simulink model "FirstPrincValveInjector_AlgebraicLoopOnly_Testing"  (R2025b)
settings: Solver=VariableStepAuto  StartTime=0.0  StopTime=10.0  RelTol=1e-3
undefined symbols (not defined in the file): A_inj_ox, Cd_inj_ox, CdA_table, epsilon, mdot_ox_nom_cstar_match, P_1_ox, P_c_nom, psi_to_Pa, rho_ox, theta_bp
settings Model: Creator=gruby  LastModifiedBy=gruby

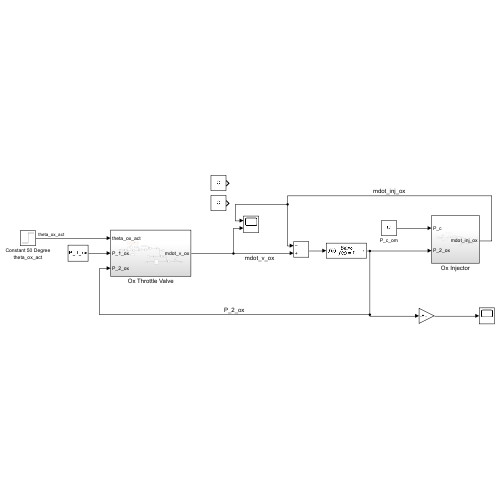
[thumbnail: Simulink's stored preview of the top-level diagram]
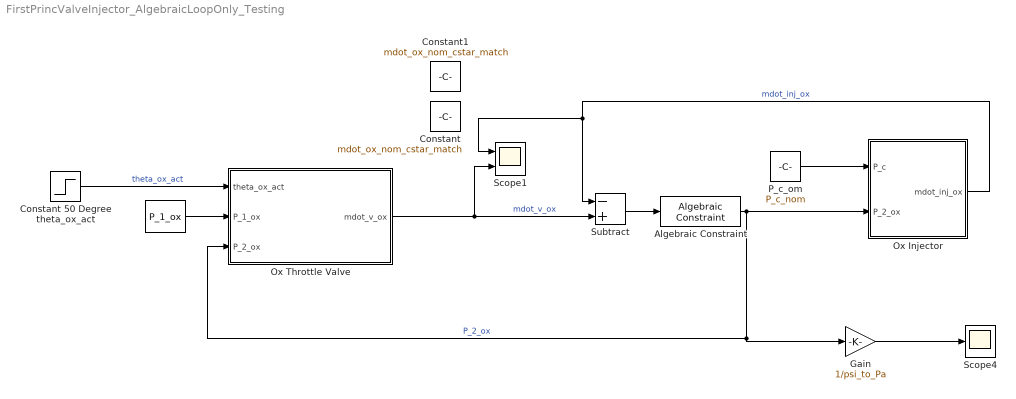
== system FirstPrincValveInjector_AlgebraicLoopOnly_Testing ==
  " " : Constant  Value=P_1_ox
  Algebraic Constraint : AlgebraicConstraint  InitialGuess=P_amb
  Constant : Constant  Value=mdot_ox_nom_cstar_match
  Constant 50 Degree theta_ox_act : Step  Time=10  Before=50  After=50  SampleTime=0
  Constant1 : Constant  Value=mdot_ox_nom_cstar_match
  Gain : Gain  Gain=1/psi_to_Pa
  Ox Injector : Subsystem
  Ox Throttle Valve : Subsystem
  P_c_om : Constant  Value=P_c_nom
  Scope1 : Scope  NumInputPorts=2
      settings: ActiveDisplayYMinimum=-1  ActiveDisplayYMaximum=1  DataLoggingVariableName=ScopeData3
  Scope4 : Scope
      settings: ActiveDisplayYMinimum=299.56325226947473  ActiveDisplayYMaximum=499.56325226947473  DataLoggingVariableName=ScopeData18
  Subtract : Sum  Inputs=-+
  wires:
  Ox Injector/1(mdot_inj_ox) -> Subtract/1, Scope1/1  "mdot_inj_ox"
  " "/1 -> Ox Throttle Valve/2(P_1_ox)
  Ox Throttle Valve/1(mdot_v_ox) -> Scope1/2, Subtract/2  "mdot_v_ox"
  Algebraic Constraint/1 -> Ox Injector/2(P_2_ox), Ox Throttle Valve/3(P_2_ox), Gain/1  "P_2_ox"
  Subtract/1 -> Algebraic Constraint/1
  Constant 50 Degree theta_ox_act/1 -> Ox Throttle Valve/1(theta_ox_act)  "theta_ox_act"
  P_c_om/1 -> Ox Injector/1(P_c)
  Gain/1 -> Scope4/1

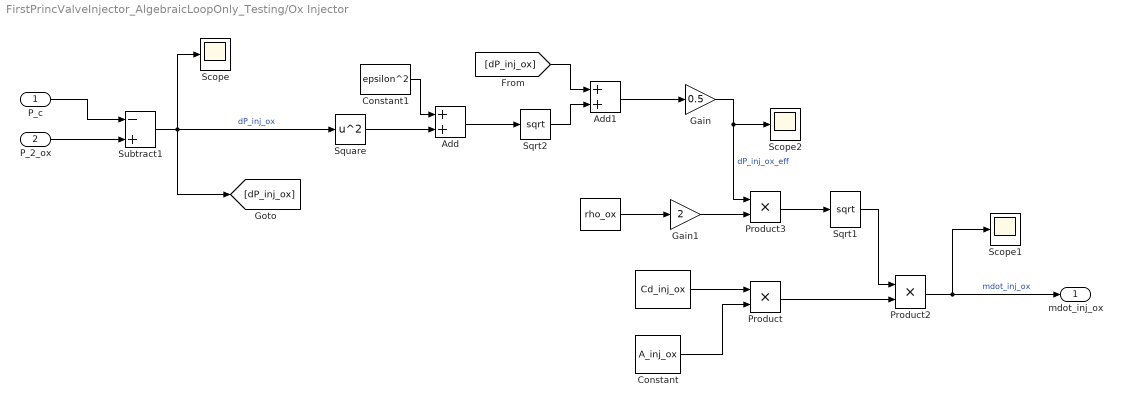
== system FirstPrincValveInjector_AlgebraicLoopOnly_Testing/Ox Injector ==
  P_c : Inport
  P_2_ox : Inport  Port=2
  " " : Constant  Value=rho_ox
  "    " : Constant  Value=Cd_inj_ox
  Add : Sum
  Add1 : Sum
  Constant : Constant  Value=A_inj_ox
  Constant1 : Constant  Value=epsilon^2
  Gain : Gain  Gain=0.5
  Gain1 : Gain  Gain=2
  Product : Product
  Product2 : Product
  Product3 : Product
  Scope : Scope
      settings: ActiveDisplayYMinimum=-1  ActiveDisplayYMaximum=1
  Scope1 : Scope
      settings: ActiveDisplayYMinimum=-1  ActiveDisplayYMaximum=1  DataLoggingVariableName=ScopeData2
  Scope2 : Scope
      settings: DataLoggingVariableName=ScopeData21
  Sqrt1 : Sqrt
  Sqrt2 : Sqrt
  Square : Math  Operator=square
  Subtract1 : Sum  Inputs=-+
  mdot_inj_ox : Outport
  wires:
  Subtract1/1 -> [dP_inj_ox], Square/1, Scope/1  "dP_inj_ox"
  "    "/1 -> Product/1
  " "/1 -> Gain1/1
  P_2_ox/1 -> Subtract1/2
  Product3/1 -> Sqrt1/1
  Sqrt1/1 -> Product2/1
  Gain1/1 -> Product3/2
  P_c/1 -> Subtract1/1
  Product2/1 -> Scope1/1, mdot_inj_ox/1  "mdot_inj_ox"
  Constant/1 -> Product/2
  Product/1 -> Product2/2
  Add1/1 -> Gain/1
  Sqrt2/1 -> Add1/2
  Add/1 -> Sqrt2/1
  [dP_inj_ox] -> Add1/1
  Constant1/1 -> Add/1
  Square/1 -> Add/2
  Gain/1 -> Product3/1, Scope2/1  "dP_inj_ox_eff"

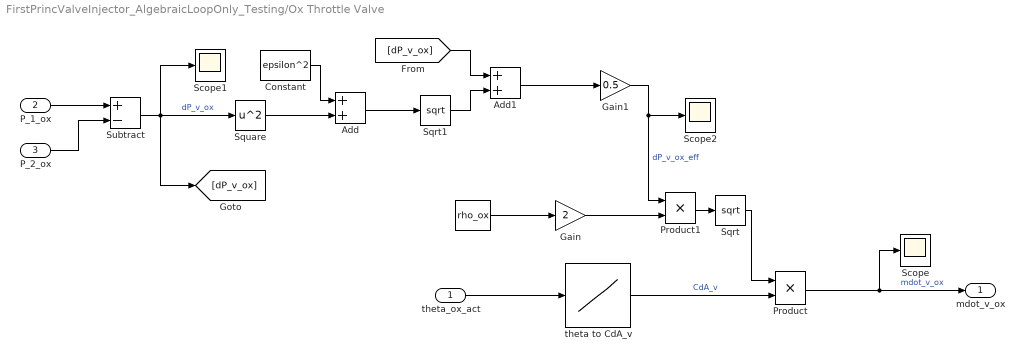
== system FirstPrincValveInjector_AlgebraicLoopOnly_Testing/Ox Throttle Valve ==
  theta_ox_act : Inport
  P_1_ox : Inport  Port=2
  P_2_ox : Inport  Port=3
  "  " : Constant  Value=rho_ox
  Add : Sum
  Add1 : Sum
  Constant : Constant  Value=epsilon^2
  Gain : Gain  Gain=2
  Gain1 : Gain  Gain=0.5
  Product : Product
  Product1 : Product
  Scope : Scope
      settings: ActiveDisplayYMinimum=-1  ActiveDisplayYMaximum=1  DataLoggingVariableName=ScopeData6
  Scope1 : Scope
      settings: ActiveDisplayYMinimum=-1  ActiveDisplayYMaximum=1  DataLoggingVariableName=ScopeData10
  Scope2 : Scope
      settings: ActiveDisplayYMinimum=-1  ActiveDisplayYMaximum=1  DataLoggingVariableName=ScopeData19
  Sqrt : Sqrt
  Sqrt1 : Sqrt
  Square : Math  Operator=square
  Subtract : Sum  Inputs=+-
  theta to CdA_v : Lookup_n-D  NumberOfTableDimensions=1  BreakpointsForDimension1=theta_bp  Table=CdA_table  ExtrapMethod=Clip  UseLastTableValue=on  InternalRulePriority=Speed  RndMeth=Simplest
  mdot_v_ox : Outport
  wires:
  Subtract/1 -> [dP_v_ox], Square/1, Scope1/1  "dP_v_ox"
  Sqrt/1 -> Product/1
  "  "/1 -> Gain/1
  Product/1 -> Scope/1, mdot_v_ox/1  "mdot_v_ox"
  Gain/1 -> Product1/2
  theta to CdA_v/1 -> Product/2  "CdA_v"
  Product1/1 -> Sqrt/1
  theta_ox_act/1 -> theta to CdA_v/1
  P_1_ox/1 -> Subtract/1
  P_2_ox/1 -> Subtract/2
  Square/1 -> Add/2
  Constant/1 -> Add/1
  Add/1 -> Sqrt1/1
  [dP_v_ox] -> Add1/1
  Sqrt1/1 -> Add1/2
  Add1/1 -> Gain1/1
  Gain1/1 -> Product1/1, Scope2/1  "dP_v_ox_eff"
